simulink model "ControlePD_ind_pos"  (R2020a)
settings: Solver=FixedStepAuto  StartTime=0.0  StopTime=10  FixedStep=Ts
values from neighbouring files (symbols this model uses):
  Beff = 50    [controle.m]    (also in controle_FF.m; controle_PD.m)
  Jeff = 2.2    [controle.m]    (also in controle_FF.m = 0.5; controle_PD.m = 0.5)
  K = 17.7    [controle.m]    (also in controle_FF.m = 0.785398163397; controle_PD.m = 0.785398163397)
  Kd = (2*zeta*wn*Jeff - Beff)/K    (= -2.32768361582)    [controle.m]    (also in controle_FF.m = -44.5633840657; controle_PD.m = -44.5633840657)
  Kp = (wn^2*Jeff)/K    (= 0.497175141243)    [controle.m]    (also in controle_FF.m = 143.239448783; controle_PD.m = 143.239448783)
  N = 10    [controle.m]    (also in controle_FF.m = 3; controle_PD.m = 3)
  r = 1/100    (= 0.01)    [controle.m]    (also in controle_FF.m = 1./[231.22*4 139.138 139.138 231.22 231.22]; controle_PD.m = 1./[231.22*4 139.138 139.138 231.22 231.22])
  SP_theta = [0;0;0;0;0]    [controle.m]    (also in controle_FF.m = [0 0 0 0 0]; controle_PD.m)
settings Model: Creator=Karoline  LastModifiedBy=lunet
settings DataIOCC: ReturnWorkspaceOutputs=off
settings DebuggingCC: ArithmeticOperatorsInVariantConditions=warning
settings SFSimCC: SimUseLocalCustomCode=off  CustomCodeUndefinedFunction=UseInterfaceOnly
settings RTWCC: RTWUseLocalCustomCode=off
settings CodeAppCC: StateflowObjectComments=on

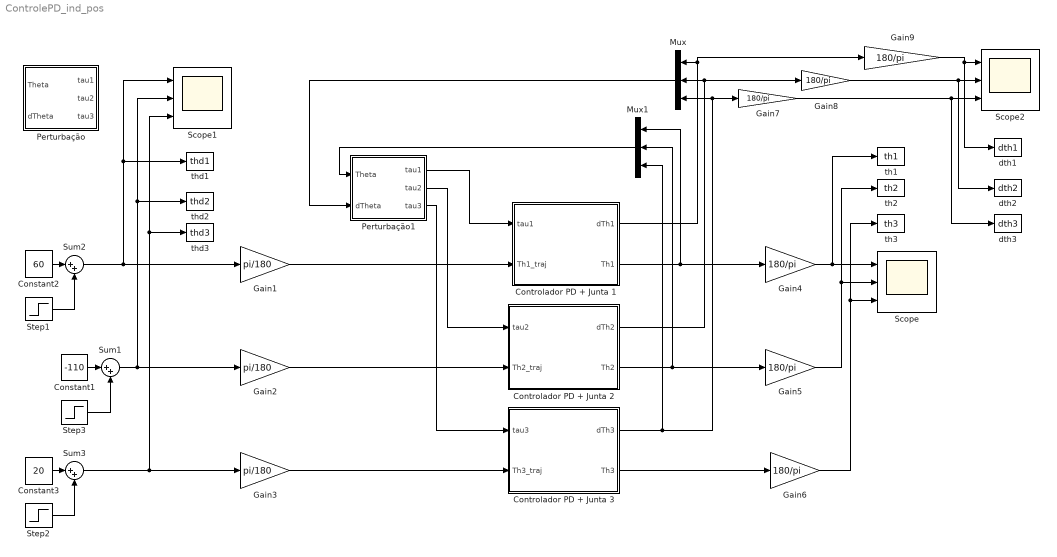
== system ControlePD_ind_pos ==
  Constant1 : Constant  Value=-110
  Constant2 : Constant  Value=60
  Constant3 : Constant  Value=20
  Controlador PD + Junta 1 : Subsystem
  Controlador PD + Junta 2 : Subsystem
  Controlador PD + Junta 3 : Subsystem
  Gain1 : Gain  Gain=pi/180
  Gain2 : Gain  Gain=pi/180
  Gain3 : Gain  Gain=pi/180
  Gain{4..9} (6 alike) : Gain  Gain=180/pi
  Mux : Mux  Inputs=3
  Mux1 : Mux  Inputs=3
  Perturbação : Subsystem
  Perturbação1 : Subsystem
  Scope : Scope  NumInputPorts=3
  Scope1 : Scope  NumInputPorts=3
  Scope2 : Scope  NumInputPorts=3
  Step1 : Step  Time=0  After=0  SampleTime=0
  Step2 : Step  Time=0  After=0  SampleTime=0
  Step3 : Step  Time=3  After=60  SampleTime=0
  Sum1 : Sum  Inputs=|++
  Sum2 : Sum  Inputs=|++
  Sum3 : Sum  Inputs=|++
  dth1 : ToWorkspace  VariableName=dth1  SampleTime=-1
  dth2 : ToWorkspace  VariableName=dth2  SampleTime=-1
  dth3 : ToWorkspace  VariableName=dth3  SampleTime=-1
  th1 : ToWorkspace  VariableName=th1  SampleTime=-1
  th2 : ToWorkspace  VariableName=th2  SampleTime=-1
  th3 : ToWorkspace  VariableName=th3  SampleTime=-1
  thd1 : ToWorkspace  VariableName=thd1  SampleTime=-1
  "thd2 " : ToWorkspace  VariableName=thd2  SampleTime=-1
  thd3 : ToWorkspace  VariableName=thd3  SampleTime=-1
  wires:
  Sum2/1 -> thd1/1, Scope1/1, Gain1/1
  Mux/1 -> Perturbação1/2(dTheta)
  Mux1/1 -> Perturbação1/1(Theta)
  Sum3/1 -> Scope1/3, thd3/1, Gain3/1
  Step3/1 -> Sum1/2
  Sum1/1 -> Scope1/2, "thd2 "/1, Gain2/1
  Constant1/1 -> Sum1/1
  Gain1/1 -> Controlador PD + Junta 1/2(Th1_traj)
  Gain2/1 -> Controlador PD + Junta 2/2(Th2_traj)
  Gain3/1 -> Controlador PD + Junta 3/2(Th3_traj)
  Gain4/1 -> th1/1, Scope/1
  Gain5/1 -> th2/1, Scope/2
  Gain6/1 -> th3/1, Scope/3
  Controlador PD + Junta 1/1("dTh1 ") -> Mux/1, Gain9/1
  Controlador PD + Junta 2/1("dTh2 ") -> Mux/2, Gain8/1
  Controlador PD + Junta 3/1("dTh3 ") -> Mux1/3, Mux/3, Gain7/1
  Controlador PD + Junta 1/2(Th1) -> Mux1/1, Gain4/1
  Controlador PD + Junta 2/2(Th2) -> Mux1/2, Gain5/1
  Controlador PD + Junta 3/2(Th3) -> Gain6/1
  Gain7/1 -> dth3/1, Scope2/3
  Gain8/1 -> dth2/1, Scope2/2
  Gain9/1 -> dth1/1, Scope2/1
  Step1/1 -> Sum2/2
  Constant2/1 -> Sum2/1
  Step2/1 -> Sum3/2
  Constant3/1 -> Sum3/1
  Perturbação1/1(tau1) -> Controlador PD + Junta 1/1(tau1)
  Perturbação1/2(tau2) -> Controlador PD + Junta 2/1(tau2)
  Perturbação1/3(tau3) -> Controlador PD + Junta 3/1(tau3)

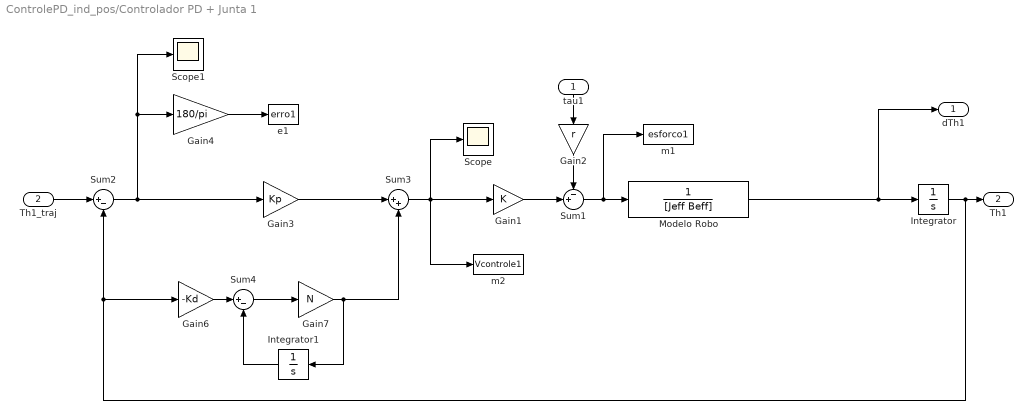
== system ControlePD_ind_pos/Controlador PD + Junta 1 ==
  tau1 : Inport
  Th1_traj : Inport  Port=2
  Gain1 : Gain  Gain=K
  Gain2 : Gain  Gain=r
  Gain3 : Gain  Gain=Kp
  Gain4 : Gain  Gain=180/pi
  Gain6 : Gain  Gain=-Kd
  Gain7 : Gain  Gain=N
  Integrator : Integrator  InitialCondition=SP_theta(1)*pi/180
  Integrator1 : Integrator
  Modelo Robo : TransferFcn  Denominator=[Jeff Beff]
  Scope : Scope
  Scope1 : Scope
  Sum1 : Sum  Inputs=-+|
  Sum2 : Sum  Inputs=|+-
  Sum3 : Sum  Inputs=|++
  Sum4 : Sum  Inputs=|+-
  e1 : ToWorkspace  VariableName=erro1  SampleTime=-1
  m1 : ToWorkspace  VariableName=esforco1  SampleTime=-1
  m2 : ToWorkspace  VariableName=Vcontrole1  SampleTime=-1
  "dTh1 " : Outport  VectorParamsAs1DForOutWhenUnconnected=off
  Th1 : Outport  Port=2  VectorParamsAs1DForOutWhenUnconnected=off
  wires:
  tau1/1 -> Gain2/1
  Gain1/1 -> Sum1/2
  Sum1/1 -> m1/1, Modelo Robo/1
  Integrator/1 -> Th1/1, Gain6/1, Sum2/2
  Th1_traj/1 -> Sum2/1
  Gain2/1 -> Sum1/1
  Gain4/1 -> e1/1
  Gain3/1 -> Sum3/1
  Sum3/1 -> m2/1, Scope/1, Gain1/1
  Modelo Robo/1 -> "dTh1 "/1, Integrator/1
  Gain7/1 -> Sum3/2, Integrator1/1
  Integrator1/1 -> Sum4/2
  Gain6/1 -> Sum4/1
  Sum4/1 -> Gain7/1
  Sum2/1 -> Gain3/1, Scope1/1, Gain4/1

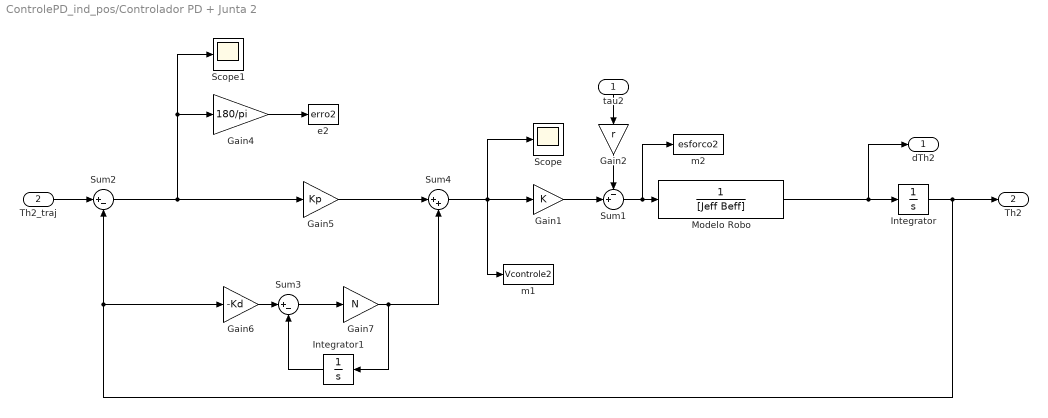
== system ControlePD_ind_pos/Controlador PD + Junta 2 ==
  tau2 : Inport
  Th2_traj : Inport  Port=2
  Gain1 : Gain  Gain=K
  Gain2 : Gain  Gain=r
  Gain4 : Gain  Gain=180/pi
  Gain5 : Gain  Gain=Kp
  Gain6 : Gain  Gain=-Kd
  Gain7 : Gain  Gain=N
  Integrator : Integrator  InitialCondition=SP_theta(2)*pi/180
  Integrator1 : Integrator
  "Modelo Robo " : TransferFcn  Denominator=[Jeff Beff]
  Scope : Scope
  Scope1 : Scope
  Sum1 : Sum  Inputs=-+|
  Sum2 : Sum  Inputs=|+-
  Sum3 : Sum  Inputs=|+-
  Sum4 : Sum  Inputs=|++
  e2 : ToWorkspace  VariableName=erro2  SampleTime=-1
  m1 : ToWorkspace  VariableName=Vcontrole2  SampleTime=-1
  m2 : ToWorkspace  VariableName=esforco2  SampleTime=-1
  "dTh2 " : Outport  VectorParamsAs1DForOutWhenUnconnected=off
  Th2 : Outport  Port=2  VectorParamsAs1DForOutWhenUnconnected=off
  wires:
  tau2/1 -> Gain2/1
  Gain1/1 -> Sum1/2
  Sum1/1 -> m2/1, "Modelo Robo "/1
  Th2_traj/1 -> Sum2/1
  Gain2/1 -> Sum1/1
  Gain4/1 -> e2/1
  Gain5/1 -> Sum4/1
  Sum4/1 -> m1/1, Scope/1, Gain1/1
  "Modelo Robo "/1 -> "dTh2 "/1, Integrator/1
  Sum2/1 -> Scope1/1, Gain4/1, Gain5/1
  Integrator1/1 -> Sum3/2
  Gain7/1 -> Sum4/2, Integrator1/1
  Integrator/1 -> Th2/1, Gain6/1, Sum2/2
  Sum3/1 -> Gain7/1
  Gain6/1 -> Sum3/1

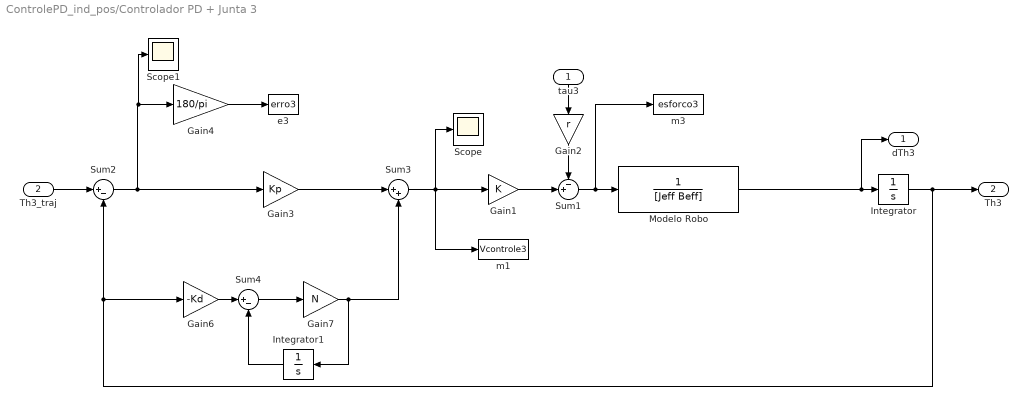
== system ControlePD_ind_pos/Controlador PD + Junta 3 ==
  tau3 : Inport
  Th3_traj : Inport  Port=2
  Gain1 : Gain  Gain=K
  Gain2 : Gain  Gain=r
  Gain3 : Gain  Gain=Kp
  Gain4 : Gain  Gain=180/pi
  Gain6 : Gain  Gain=-Kd
  Gain7 : Gain  Gain=N
  Integrator : Integrator  InitialCondition=SP_theta(3)*pi/180
  Integrator1 : Integrator
  Modelo Robo : TransferFcn  Denominator=[Jeff Beff]
  Scope : Scope
  Scope1 : Scope
  Sum1 : Sum  Inputs=-+|
  Sum2 : Sum  Inputs=|+-
  Sum3 : Sum  Inputs=|++
  Sum4 : Sum  Inputs=|+-
  e3 : ToWorkspace  VariableName=erro3  SampleTime=-1
  m1 : ToWorkspace  VariableName=Vcontrole3  SampleTime=-1
  m3 : ToWorkspace  VariableName=esforco3  SampleTime=-1
  "dTh3 " : Outport  VectorParamsAs1DForOutWhenUnconnected=off
  Th3 : Outport  Port=2  VectorParamsAs1DForOutWhenUnconnected=off
  wires:
  tau3/1 -> Gain2/1
  Gain1/1 -> Sum1/2
  Sum1/1 -> m3/1, Modelo Robo/1
  Th3_traj/1 -> Sum2/1
  Gain2/1 -> Sum1/1
  Gain4/1 -> e3/1
  Gain3/1 -> Sum3/1
  Sum3/1 -> m1/1, Scope/1, Gain1/1
  Modelo Robo/1 -> Integrator/1, "dTh3 "/1
  Sum2/1 -> Scope1/1, Gain4/1, Gain3/1
  Integrator1/1 -> Sum4/2
  Gain7/1 -> Sum3/2, Integrator1/1
  Integrator/1 -> Th3/1, Gain6/1, Sum2/2
  Sum4/1 -> Gain7/1
  Gain6/1 -> Sum4/1

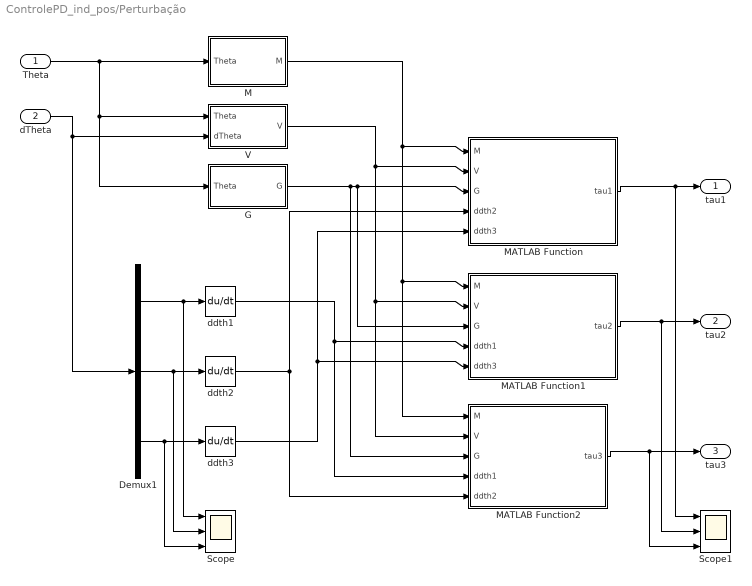
== system ControlePD_ind_pos/Perturbação ==
  Theta : Inport
  dTheta : Inport  Port=2
  Demux1 : Demux  Outputs=3
  G : Subsystem
  M : Subsystem
  MATLAB Function : MATLAB Function  TreatAsAtomicUnit=on
  MATLAB Function1 : MATLAB Function  TreatAsAtomicUnit=on
  MATLAB Function2 : MATLAB Function  TreatAsAtomicUnit=on
  Scope : Scope  NumInputPorts=3
  Scope1 : Scope  NumInputPorts=3
  V : Subsystem
  ddth1 : Derivative
  ddth2 : Derivative
  ddth3 : Derivative
  tau1 : Outport  VectorParamsAs1DForOutWhenUnconnected=off
  tau2 : Outport  Port=2  VectorParamsAs1DForOutWhenUnconnected=off
  tau3 : Outport  Port=3  VectorParamsAs1DForOutWhenUnconnected=off
  wires:
  dTheta/1 -> Demux1/1, V/2(dTheta)
  G/1(G) -> MATLAB Function2/3(G), MATLAB Function1/3(G), MATLAB Function/3(G)
  V/1(V) -> MATLAB Function/2(V), MATLAB Function1/2(V), MATLAB Function2/2(V)
  M/1(M) -> MATLAB Function2/1(M), MATLAB Function1/1(M), MATLAB Function/1(M)
  Theta/1 -> M/1(Theta), G/1(Theta), V/1(Theta)
  Demux1/1 -> Scope/1, ddth1/1
  Demux1/2 -> Scope/2, ddth2/1
  Demux1/3 -> Scope/3, ddth3/1
  ddth1/1 -> MATLAB Function2/4(ddth1), MATLAB Function1/4(ddth1)
  ddth3/1 -> MATLAB Function/5(ddth3), MATLAB Function1/5(ddth3)
  ddth2/1 -> MATLAB Function2/5(ddth2), MATLAB Function/4(ddth2)
  MATLAB Function/1(tau1) -> Scope1/1, tau1/1
  MATLAB Function1/1(tau2) -> Scope1/2, tau2/1
  MATLAB Function2/1(tau3) -> Scope1/3, tau3/1

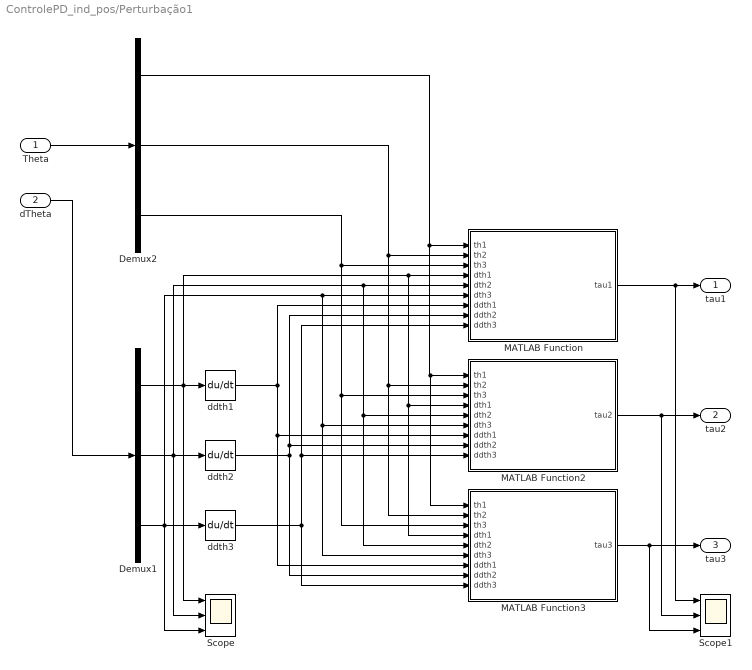
== system ControlePD_ind_pos/Perturbação1 ==
  Theta : Inport
  dTheta : Inport  Port=2
  Demux1 : Demux  Outputs=3
  Demux2 : Demux  Outputs=3
  MATLAB Function : MATLAB Function  TreatAsAtomicUnit=on
  MATLAB Function2 : MATLAB Function  TreatAsAtomicUnit=on
  MATLAB Function3 : MATLAB Function  TreatAsAtomicUnit=on
  Scope : Scope  NumInputPorts=3
  Scope1 : Scope  NumInputPorts=3
  ddth1 : Derivative
  ddth2 : Derivative
  ddth3 : Derivative
  tau1 : Outport  VectorParamsAs1DForOutWhenUnconnected=off
  tau2 : Outport  Port=2  VectorParamsAs1DForOutWhenUnconnected=off
  tau3 : Outport  Port=3  VectorParamsAs1DForOutWhenUnconnected=off
  wires:
  dTheta/1 -> Demux1/1
  Demux1/1 -> MATLAB Function3/4(dth1), MATLAB Function2/4(dth1), MATLAB Function/4(dth1), Scope/1, ddth1/1
  Demux1/2 -> MATLAB Function3/5(dth2), MATLAB Function2/5(dth2), MATLAB Function/5(dth2), Scope/2, ddth2/1
  Demux1/3 -> MATLAB Function3/6(dth3), MATLAB Function2/6(dth3), MATLAB Function/6(dth3), Scope/3, ddth3/1
  ddth1/1 -> MATLAB Function3/7(ddth1), MATLAB Function2/7(ddth1), MATLAB Function/7(ddth1)
  ddth3/1 -> MATLAB Function3/9(ddth3), MATLAB Function2/9(ddth3), MATLAB Function/9(ddth3)
  ddth2/1 -> MATLAB Function3/8(ddth2), MATLAB Function2/8(ddth2), MATLAB Function/8(ddth2)
  MATLAB Function/1(tau1) -> tau1/1, Scope1/1
  MATLAB Function2/1(tau2) -> tau2/1, Scope1/2
  MATLAB Function3/1(tau3) -> tau3/1, Scope1/3
  Theta/1 -> Demux2/1
  Demux2/3 -> MATLAB Function3/3(th3), MATLAB Function2/3(th3), MATLAB Function/3(th3)
  Demux2/2 -> MATLAB Function3/2(th2), MATLAB Function2/2(th2), MATLAB Function/2(th2)
  Demux2/1 -> MATLAB Function3/1(th1), MATLAB Function2/1(th1), MATLAB Function/1(th1)

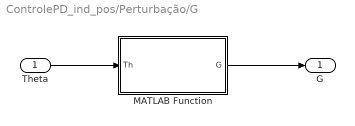
== system ControlePD_ind_pos/Perturbação/G ==
  Theta : Inport
  MATLAB Function : MATLAB Function  TreatAsAtomicUnit=on
  G : Outport  VectorParamsAs1DForOutWhenUnconnected=off
  wires:
  Theta/1 -> MATLAB Function/1(Th)
  MATLAB Function/1(G) -> G/1

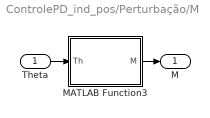
== system ControlePD_ind_pos/Perturbação/M ==
  Theta : Inport
  MATLAB Function3 : MATLAB Function  TreatAsAtomicUnit=on
  M : Outport  VectorParamsAs1DForOutWhenUnconnected=off
  wires:
  Theta/1 -> MATLAB Function3/1(Th)
  MATLAB Function3/1(M) -> M/1

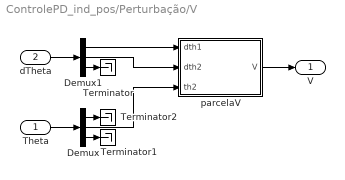
== system ControlePD_ind_pos/Perturbação/V ==
  Theta : Inport
  dTheta : Inport  Port=2
  Demux : Demux  Outputs=3
  Demux1 : Demux  Outputs=3
  Terminator : Terminator
  Terminator1 : Terminator
  Terminator2 : Terminator
  parcelaV : MATLAB Function  TreatAsAtomicUnit=on
  V : Outport  VectorParamsAs1DForOutWhenUnconnected=off
  wires:
  Theta/1 -> Demux/1
  dTheta/1 -> Demux1/1
  Demux1/1 -> parcelaV/1(dth1)
  Demux1/2 -> parcelaV/2(dth2)
  Demux/2 -> parcelaV/3(th2)
  parcelaV/1(V) -> V/1
  Demux1/3 -> Terminator/1
  Demux/1 -> Terminator2/1
  Demux/3 -> Terminator1/1

== matlab function ControlePD_ind_pos/Perturbação1/MATLAB Function ==
  data: th1 input; th2 input; tau1 output; th3 input; dth1 input; dth2 input; dth3 input; ddth1 input; ddth2 input; ddth3 input
function tau1  = calcul_dk1(th1,th2,th3,dth1,dth2,dth3,ddth1,ddth2,ddth3)

I1 = 1;
I2 = 1;
I3 = 1;
m1 = 1;
m2 = 1;
m3 = 1;
Lc1 = 0.05;
Lc2 = 0.05;
Lc3 = 0.05;
g = 9.81;

tau1 = I1*ddth1 + I2*ddth1*cos(th2)^2 + I2*ddth1*sin(th2)^2 + I3*ddth1*cos(th2)^2*cos(th3)^2 + I3*ddth1*cos(th2)^2*sin(th3)^2 + I3*ddth1*cos(th3)^2*sin(th2)^2 + I3*ddth1*sin(th2)^2*sin(th3)^2 + (ddth1*m3*cos(th1)^2*cos(th2)^2)/25 + (ddth1*m3*cos(th2)^2*sin(th1)^2)/25 + Lc2^2*ddth1*m2*cos(th1)^2*cos(th2)^2 + Lc2^2*ddth1*m2*cos(th2)^2*sin(th1)^2 - (2*dth1*dth2*m3*cos(th1)^2*cos(th2)*sin(th2))/25 + Lc3^2*ddth1*m3*cos(th1)^2*cos(th2)^2*sin(th3)^2 + Lc3^2*ddth1*m3*cos(th1)^2*cos(th3)^2*sin(th2)^2 - (2*dth1*dth2*m3*cos(th2)*sin(th1)^2*sin(th2))/25 + Lc3^2*ddth1*m3*cos(th2)^2*sin(th1)^2*sin(th3)^2 + Lc3^2*ddth1*m3*cos(th3)^2*sin(th1)^2*sin(th2)^2 - (2*Lc3*ddth1*m3*cos(th1)^2*cos(th2)^2*sin(th3))/5 - (2*Lc3*ddth1*m3*cos(th2)^2*sin(th1)^2*sin(th3))/5 - (2*Lc3*dth1*dth2*m3*cos(th1)^2*cos(th2)^2*cos(th3))/5 - (2*Lc3*dth1*dth3*m3*cos(th1)^2*cos(th2)^2*cos(th3))/5 - 2*Lc2^2*dth1*dth2*m2*cos(th1)^2*cos(th2)*sin(th2) + (2*Lc3*dth1*dth2*m3*cos(th1)^2*cos(th3)*sin(th2)^2)/5 - (2*Lc3*dth1*dth2*m3*cos(th2)^2*cos(th3)*sin(th1)^2)/5 - (2*Lc3*dth1*dth3*m3*cos(th2)^2*cos(th3)*sin(th1)^2)/5 - 2*Lc2^2*dth1*dth2*m2*cos(th2)*sin(th1)^2*sin(th2) + (2*Lc3*dth1*dth2*m3*cos(th3)*sin(th1)^2*sin(th2)^2)/5 - (2*Lc3*ddth1*m3*cos(th1)^2*cos(th2)*cos(th3)*sin(th2))/5 - (2*Lc3*ddth1*m3*cos(th2)*cos(th3)*sin(th1)^2*sin(th2))/5 + 2*Lc3^2*dth1*dth2*m3*cos(th1)^2*cos(th2)*cos(th3)^2*sin(th2) + 2*Lc3^2*dth1*dth2*m3*cos(th1)^2*cos(th2)^2*cos(th3)*sin(th3) + 2*Lc3^2*dth1*dth3*m3*cos(th1)^2*cos(th2)*cos(th3)^2*sin(th2) + 2*Lc3^2*dth1*dth3*m3*cos(th1)^2*cos(th2)^2*cos(th3)*sin(th3) + 2*Lc3^2*dth1*dth2*m3*cos(th2)*cos(th3)^2*sin(th1)^2*sin(th2) - 2*Lc3^2*dth1*dth2*m3*cos(th1)^2*cos(th2)*sin(th2)*sin(th3)^2 - 2*Lc3^2*dth1*dth2*m3*cos(th1)^2*cos(th3)*sin(th2)^2*sin(th3) + 2*Lc3^2*dth1*dth2*m3*cos(th2)^2*cos(th3)*sin(th1)^2*sin(th3) + 2*Lc3^2*dth1*dth3*m3*cos(th2)*cos(th3)^2*sin(th1)^2*sin(th2) - 2*Lc3^2*dth1*dth3*m3*cos(th1)^2*cos(th2)*sin(th2)*sin(th3)^2 - 2*Lc3^2*dth1*dth3*m3*cos(th1)^2*cos(th3)*sin(th2)^2*sin(th3) + 2*Lc3^2*dth1*dth3*m3*cos(th2)^2*cos(th3)*sin(th1)^2*sin(th3) - 2*Lc3^2*dth1*dth2*m3*cos(th2)*sin(th1)^2*sin(th2)*sin(th3)^2 - 2*Lc3^2*dth1*dth2*m3*cos(th3)*sin(th1)^2*sin(th2)^2*sin(th3) - 2*Lc3^2*dth1*dth3*m3*cos(th2)*sin(th1)^2*sin(th2)*sin(th3)^2 - 2*Lc3^2*dth1*dth3*m3*cos(th3)*sin(th1)^2*sin(th2)^2*sin(th3) + 2*Lc3^2*ddth1*m3*cos(th1)^2*cos(th2)*cos(th3)*sin(th2)*sin(th3) + 2*Lc3^2*ddth1*m3*cos(th2)*cos(th3)*sin(th1)^2*sin(th2)*sin(th3) + (4*Lc3*dth1*dth2*m3*cos(th1)^2*cos(th2)*sin(th2)*sin(th3))/5 + (2*Lc3*dth1*dth3*m3*cos(th1)^2*cos(th2)*sin(th2)*sin(th3))/5 + (4*Lc3*dth1*dth2*m3*cos(th2)*sin(th1)^2*sin(th2)*sin(th3))/5 + (2*Lc3*dth1*dth3*m3*cos(th2)*sin(th1)^2*sin(th2)*sin(th3))/5;

== matlab function ControlePD_ind_pos/Perturbação1/MATLAB Function2 ==
  data: th1 input; th2 input; tau2 output; th3 input; dth1 input; dth2 input; dth3 input; ddth1 input; ddth2 input; ddth3 input
function tau2  = calcul_dk2(th1,th2,th3,dth1,dth2,dth3,ddth1,ddth2,ddth3)

I1 = 1;
I2 = 1;
I3 = 1;
m1 = 1;
m2 = 1;
m3 = 1;
Lc1 = 0.05;
Lc2 = 0.05;
Lc3 = 0.05;
g = 9.81;

tau2 =   I2*ddth2 + I3*ddth2 + I3*ddth3 + Lc2^2*ddth2*m2*cos(th2)^2 - Lc3*g*m3*sin(th2 + th3) + Lc2*g*m2*cos(th2) + (ddth2*m3*cos(th2 + th3)^2*cos(th3)^2)/25 + (ddth2*m3*sin(th2 + th3)^2*sin(th3)^2)/25 + Lc3^2*ddth2*m3*sin(th2 + th3)^2 + Lc3^2*ddth3*m3*sin(th2 + th3)^2 + Lc3^2*ddth2*m3*cos(th2 + th3)^2*cos(th1)^2 + Lc3^2*ddth3*m3*cos(th2 + th3)^2*cos(th1)^2 - (dth2^2*m3*cos(th2 + th3)*sin(th2 + th3)*cos(th3)^2)/25 + Lc3^2*ddth2*m3*cos(th2 + th3)^2*sin(th1)^2 + Lc3^2*ddth3*m3*cos(th2 + th3)^2*sin(th1)^2 + (dth2^2*m3*cos(th2 + th3)*sin(th2 + th3)*sin(th3)^2)/25 + (dth2^2*m3*cos(th2 + th3)^2*cos(th3)*sin(th3))/25 + Lc2^2*ddth2*m2*cos(th1)^2*sin(th2)^2 - (dth2^2*m3*sin(th2 + th3)^2*cos(th3)*sin(th3))/25 + Lc2^2*ddth2*m2*sin(th1)^2*sin(th2)^2 - (2*Lc3*ddth2*m3*sin(th2 + th3)^2*sin(th3))/5 - (Lc3*ddth3*m3*sin(th2 + th3)^2*sin(th3))/5 - (dth1^2*m3*cos(th1)^2*cos(th2)*sin(th2))/25 - (dth1^2*m3*cos(th2)*sin(th1)^2*sin(th2))/25 + Lc3^2*dth2^2*m3*cos(th2 + th3)*sin(th2 + th3) + Lc3^2*dth3^2*m3*cos(th2 + th3)*sin(th2 + th3) + (ddth2*m3*cos(th2 + th3)^2*cos(th1)^2*sin(th3)^2)/25 + (ddth2*m3*sin(th2 + th3)^2*cos(th1)^2*cos(th3)^2)/25 - (Lc3*dth2^2*m3*cos(th2 + th3)^2*cos(th3))/5 + (ddth2*m3*cos(th2 + th3)^2*sin(th1)^2*sin(th3)^2)/25 + (ddth2*m3*sin(th2 + th3)^2*cos(th3)^2*sin(th1)^2)/25 + (Lc3*dth2^2*m3*sin(th2 + th3)^2*cos(th3))/5 - (Lc3*dth3^2*m3*sin(th2 + th3)^2*cos(th3))/5 - 3*Lc2^2*dth2^2*m2*cos(th2)*sin(th2) + (Lc3*dth2^2*m3*cos(th2 + th3)^2*cos(th3)*sin(th1)^2)/5 - (Lc3*dth2^2*m3*sin(th2 + th3)^2*cos(th1)^2*cos(th3))/5 - (Lc3*dth3^2*m3*cos(th2 + th3)^2*cos(th3)*sin(th1)^2)/5 + (2*dth2*m3*cos(th2 + th3)*sin(th2 + th3)*sin(th3)^2*(dth2 + dth3))/25 - (Lc3*dth2^2*m3*sin(th2 + th3)^2*cos(th3)*sin(th1)^2)/5 - (Lc3*dth1^2*m3*cos(th1)^2*cos(th2)^2*cos(th3))/5 + (2*dth2*m3*cos(th2 + th3)^2*cos(th3)*sin(th3)*(dth2 + dth3))/25 - (2*Lc3*dth2^2*m3*cos(th2 + th3)*sin(th2 + th3)*sin(th3))/5 + (Lc3*dth3^2*m3*cos(th2 + th3)*sin(th2 + th3)*sin(th3))/5 - Lc2^2*dth1^2*m2*cos(th1)^2*cos(th2)*sin(th2) + 3*Lc2^2*dth2^2*m2*cos(th1)^2*cos(th2)*sin(th2) + (Lc3*dth1^2*m3*cos(th1)^2*cos(th3)*sin(th2)^2)/5 - (Lc3*dth1^2*m3*cos(th2)^2*cos(th3)*sin(th1)^2)/5 + (2*dth2*dth3*m3*cos(th2 + th3)*sin(th2 + th3)*cos(th3)^2)/25 - (2*dth2*m3*sin(th2 + th3)^2*cos(th3)*sin(th3)*(dth2 + dth3))/25 - Lc2^2*dth1^2*m2*cos(th2)*sin(th1)^2*sin(th2) + 3*Lc2^2*dth2^2*m2*cos(th2)*sin(th1)^2*sin(th2) + (Lc3*dth1^2*m3*cos(th3)*sin(th1)^2*sin(th2)^2)/5 - (2*dth2*dth3*m3*cos(th2 + th3)*sin(th2 + th3)*sin(th3)^2)/25 + (2*ddth2*m3*cos(th2 + th3)*sin(th2 + th3)*cos(th3)*sin(th3))/25 - (2*dth2*dth3*m3*cos(th2 + th3)^2*cos(th3)*sin(th3))/25 + (dth2^2*m3*cos(th2 + th3)*sin(th2 + th3)*cos(th1)^2*cos(th3)^2)/25 + 2*Lc3^2*dth2*m3*cos(th2 + th3)*sin(th2 + th3)*(dth2 + dth3) + 2*Lc3^2*dth3*m3*cos(th2 + th3)*sin(th2 + th3)*(dth2 + dth3) + (2*dth2*dth3*m3*sin(th2 + th3)^2*cos(th3)*sin(th3))/25 - (dth2^2*m3*cos(th2 + th3)*sin(th2 + th3)*cos(th1)^2*sin(th3)^2)/25 + (dth2^2*m3*cos(th2 + th3)*sin(th2 + th3)*cos(th3)^2*sin(th1)^2)/25 - (dth2^2*m3*cos(th2 + th3)*sin(th2 + th3)*sin(th1)^2*sin(th3)^2)/25 - (2*Lc3*dth2*m3*cos(th2 + th3)^2*cos(th3)*(dth2 + dth3))/5 - (Lc3*dth3*m3*cos(th2 + th3)^2*cos(th3)*(dth2 + dth3))/5 - (dth2^2*m3*cos(th2 + th3)^2*cos(th1)^2*cos(th3)*sin(th3))/25 + (2*Lc3*dth2*m3*sin(th2 + th3)^2*cos(th3)*(dth2 + dth3))/5 + (Lc3*dth3*m3*sin(th2 + th3)^2*cos(th3)*(dth2 + dth3))/5 - (dth2^2*m3*cos(th2 + th3)^2*cos(th3)*sin(th1)^2*sin(th3))/25 + (dth2^2*m3*sin(th2 + th3)^2*cos(th1)^2*cos(th3)*sin(th3))/25 - (2*Lc3*ddth2*m3*cos(th2 + th3)^2*cos(th1)^2*sin(th3))/5 - (Lc3*ddth3*m3*cos(th2 + th3)^2*cos(th1)^2*sin(th3))/5 + 2*Lc3^2*dth2*dth3*m3*cos(th2 + th3)*sin(th2 + th3) + (dth2^2*m3*sin(th2 + th3)^2*cos(th3)*sin(th1)^2*sin(th3))/25 - (2*Lc3*ddth2*m3*cos(th2 + th3)^2*sin(th1)^2*sin(th3))/5 - (Lc3*ddth3*m3*cos(th2 + th3)^2*sin(th1)^2*sin(th3))/5 - (2*Lc3*ddth2*m3*cos(th2 + th3)*sin(th2 + th3)*cos(th3))/5 - (Lc3*ddth3*m3*cos(th2 + th3)*sin(th2 + th3)*cos(th3))/5 - (Lc3*dth2*dth3*m3*cos(th2 + th3)^2*cos(th3))/5 - (Lc3*dth2*dth3*m3*sin(th2 + th3)^2*cos(th3))/5 - Lc3^2*dth2^2*m3*cos(th2 + th3)*sin(th2 + th3)*cos(th1)^2 - Lc3^2*dth3^2*m3*cos(th2 + th3)*sin(th2 + th3)*cos(th1)^2 - Lc3^2*dth2^2*m3*cos(th2 + th3)*sin(th2 + th3)*sin(th1)^2 - Lc3^2*dth3^2*m3*cos(th2 + th3)*sin(th2 + th3)*sin(th1)^2 + (Lc3*dth2^2*m3*cos(th2 + th3)^2*cos(th1)^2*cos(th3))/5 - (Lc3*dth3^2*m3*cos(th2 + th3)^2*cos(th1)^2*cos(th3))/5 - (2*dth2*m3*cos(th2 + th3)*sin(th2 + th3)*cos(th3)^2*(dth2 + dth3))/25 + (2*Lc3*ddth2*m3*cos(th2 + th3)*sin(th2 + th3)*cos(th3)*sin(th1)^2)/5 + (Lc3*ddth3*m3*cos(th2 + th3)*sin(th2 + th3)*cos(th3)*sin(th1)^2)/5 - (Lc3*dth2*dth3*m3*cos(th2 + th3)^2*cos(th3)*sin(th1)^2)/5 - (Lc3*dth2*dth3*m3*sin(th2 + th3)^2*cos(th1)^2*cos(th3))/5 - (Lc3*dth2*dth3*m3*sin(th2 + th3)^2*cos(th3)*sin(th1)^2)/5 + (2*dth2*m3*cos(th2 + th3)*sin(th2 + th3)*cos(th1)^2*cos(th3)^2*(dth2 + dth3))/25 - (2*dth2*m3*cos(th2 + th3)*sin(th2 + th3)*cos(th1)^2*sin(th3)^2*(dth2 + dth3))/25 + (2*dth2*m3*cos(th2 + th3)*sin(th2 + th3)*cos(th3)^2*sin(th1)^2*(dth2 + dth3))/25 - (2*dth2*m3*cos(th2 + th3)*sin(th2 + th3)*sin(th1)^2*sin(th3)^2*(dth2 + dth3))/25 - (2*dth2*m3*cos(th2 + th3)^2*cos(th1)^2*cos(th3)*sin(th3)*(dth2 + dth3))/25 + (2*Lc3*dth2^2*m3*cos(th2 + th3)*sin(th2 + th3)*cos(th1)^2*sin(th3))/5 - (Lc3*dth3^2*m3*cos(th2 + th3)*sin(th2 + th3)*cos(th1)^2*sin(th3))/5 + Lc3^2*dth1^2*m3*cos(th1)^2*cos(th2)*cos(th3)^2*sin(th2) + Lc3^2*dth1^2*m3*cos(th1)^2*cos(th2)^2*cos(th3)*sin(th3) - (2*dth2*dth3*m3*cos(th2 + th3)*sin(th2 + th3)*cos(th1)^2*cos(th3)^2)/25 - (2*dth2*m3*cos(th2 + th3)^2*cos(th3)*sin(th1)^2*sin(th3)*(dth2 + dth3))/25 + (2*dth2*m3*sin(th2 + th3)^2*cos(th1)^2*cos(th3)*sin(th3)*(dth2 + dth3))/25 + (2*Lc3*dth2^2*m3*cos(th2 + th3)*sin(th2 + th3)*sin(th1)^2*sin(th3))/5 - (Lc3*dth3^2*m3*cos(th2 + th3)*sin(th2 + th3)*sin(th1)^2*sin(th3))/5 + Lc3^2*dth1^2*m3*cos(th2)*cos(th3)^2*sin(th1)^2*sin(th2) - Lc3^2*dth1^2*m3*cos(th1)^2*cos(th2)*sin(th2)*sin(th3)^2 - Lc3^2*dth1^2*m3*cos(th1)^2*cos(th3)*sin(th2)^2*sin(th3) + Lc3^2*dth1^2*m3*cos(th2)^2*cos(th3)*sin(th1)^2*sin(th3) + (2*dth2*dth3*m3*cos(th2 + th3)*sin(th2 + th3)*cos(th1)^2*sin(th3)^2)/25 - (2*dth2*dth3*m3*cos(th2 + th3)*sin(th2 + th3)*cos(th3)^2*sin(th1)^2)/25 + (2*dth2*m3*sin(th2 + th3)^2*cos(th3)*sin(th1)^2*sin(th3)*(dth2 + dth3))/25 - Lc3^2*dth1^2*m3*cos(th2)*sin(th1)^2*sin(th2)*sin(th3)^2 - Lc3^2*dth1^2*m3*cos(th3)*sin(th1)^2*sin(th2)^2*sin(th3) + (2*dth2*dth3*m3*cos(th2 + th3)*sin(th2 + th3)*sin(th1)^2*sin(th3)^2)/25 - (2*ddth2*m3*cos(th2 + th3)*sin(th2 + th3)*cos(th1)^2*cos(th3)*sin(th3))/25 + (2*dth2*dth3*m3*cos(th2 + th3)^2*cos(th1)^2*cos(th3)*sin(th3))/25 - (2*ddth2*m3*cos(th2 + th3)*sin(th2 + th3)*cos(th3)*sin(th1)^2*sin(th3))/25 - 2*Lc3^2*dth2*m3*cos(th2 + th3)*sin(th2 + th3)*cos(th1)^2*(dth2 + dth3) - 2*Lc3^2*dth3*m3*cos(th2 + th3)*sin(th2 + th3)*cos(th1)^2*(dth2 + dth3) + (2*dth2*dth3*m3*cos(th2 + th3)^2*cos(th3)*sin(th1)^2*sin(th3))/25 - (2*dth2*dth3*m3*sin(th2 + th3)^2*cos(th1)^2*cos(th3)*sin(th3))/25 - 2*Lc3^2*dth2*m3*cos(th2 + th3)*sin(th2 + th3)*sin(th1)^2*(dth2 + dth3) - 2*Lc3^2*dth3*m3*cos(th2 + th3)*sin(th2 + th3)*sin(th1)^2*(dth2 + dth3) - (2*dth2*dth3*m3*sin(th2 + th3)^2*cos(th3)*sin(th1)^2*sin(th3))/25 + (2*Lc3*dth1^2*m3*cos(th1)^2*cos(th2)*sin(th2)*sin(th3))/5 + (2*Lc3*dth2*m3*cos(th2 + th3)^2*cos(th1)^2*cos(th3)*(dth2 + dth3))/5 + (Lc3*dth3*m3*cos(th2 + th3)^2*cos(th1)^2*cos(th3)*(dth2 + dth3))/5 + (2*Lc3*dth1^2*m3*cos(th2)*sin(th1)^2*sin(th2)*sin(th3))/5 + (2*Lc3*dth2*m3*cos(th2 + th3)^2*cos(th3)*sin(th1)^2*(dth2 + dth3))/5 - (2*Lc3*dth2*m3*sin(th2 + th3)^2*cos(th1)^2*cos(th3)*(dth2 + dth3))/5 + (Lc3*dth3*m3*cos(th2 + th3)^2*cos(th3)*sin(th1)^2*(dth2 + dth3))/5 - (Lc3*dth3*m3*sin(th2 + th3)^2*cos(th1)^2*cos(th3)*(dth2 + dth3))/5 - 2*Lc3^2*dth2*dth3*m3*cos(th2 + th3)*sin(th2 + th3)*cos(th1)^2 - (2*Lc3*dth2*m3*sin(th2 + th3)^2*cos(th3)*sin(th1)^2*(dth2 + dth3))/5 - (Lc3*dth3*m3*sin(th2 + th3)^2*cos(th3)*sin(th1)^2*(dth2 + dth3))/5 - 2*Lc3^2*dth2*dth3*m3*cos(th2 + th3)*sin(th2 + th3)*sin(th1)^2 + (2*Lc3*ddth2*m3*cos(th2 + th3)*sin(th2 + th3)*cos(th1)^2*cos(th3))/5 + (Lc3*ddth3*m3*cos(th2 + th3)*sin(th2 + th3)*cos(th1)^2*cos(th3))/5 - (4*Lc3*dth2*m3*cos(th2 + th3)*sin(th2 + th3)*sin(th3)*(dth2 + dth3))/5 - (2*Lc3*dth3*m3*cos(th2 + th3)*sin(th2 + th3)*sin(th3)*(dth2 + dth3))/5 - (Lc3*dth2*dth3*m3*cos(th2 + th3)^2*cos(th1)^2*cos(th3))/5 + (4*Lc3*dth2*m3*cos(th2 + th3)*sin(th2 + th3)*cos(th1)^2*sin(th3)*(dth2 + dth3))/5 + (2*Lc3*dth3*m3*cos(th2 + th3)*sin(th2 + th3)*cos(th1)^2*sin(th3)*(dth2 + dth3))/5 + (4*Lc3*dth2*m3*cos(th2 + th3)*sin(th2 + th3)*sin(th1)^2*sin(th3)*(dth2 + dth3))/5 + (2*Lc3*dth3*m3*cos(th2 + th3)*sin(th2 + th3)*sin(th1)^2*sin(th3)*(dth2 + dth3))/5;

== matlab function ControlePD_ind_pos/Perturbação/G/MATLAB Function ==
  data: Th input; G output
function G = calcul_G(Th)

th1 = Th(1);
th2 = Th(2);
th3 = Th(3);

G = [(1617*cos(th1 + th2))/100 + (3871*cos(th1))/100;...
    (1617*cos(th1 + th2))/100;...
    0];

== matlab function ControlePD_ind_pos/Perturbação/MATLAB Function1 ==
  data: M input; V input; tau2 output; G input; ddth1 input; ddth3 input
function tau2  = calcul_dk2(M,V,G,ddth1, ddth3)


% tau2 = m21*ddth1 + m23*ddth3 + v2 + g2;
tau2 = M(2,1)*ddth1 + M(2,3)*ddth3 + V(2,1) + G(2);

== matlab function ControlePD_ind_pos/Perturbação/MATLAB Function ==
  data: M input; V input; tau1 output; G input; ddth2 input; ddth3 input
function tau1  = calcul_dk1(M,V,G,ddth2,ddth3)


% tau1 = m12*ddth2 + m13*ddth3 + v1 + g1;
tau1 = M(1,2)*ddth2 + M(1,3)*ddth3 + V(1,1) + G(1);

== matlab function ControlePD_ind_pos/Perturbação/MATLAB Function2 ==
  data: M input; V input; tau3 output; G input; ddth1 input; ddth2 input
function tau3  = calcul_dk3(M, V, G, ddth1, ddth2)



% tau3 = m31*ddth1 + m32*ddth2 + v3 + g3;
tau3 = M(3,1)*ddth1 + M(3,2)*ddth2 + V(3,1) + G(3);

== matlab function ControlePD_ind_pos/Perturbação/M/MATLAB Function3 ==
  data: Th input; M output
function M = calcul_M(Th)

th1 = Th(1);
th2 = Th(2);
th3 = Th(3);

M = [(33*cos(th2))/20 + 29/10, (33*cos(th2))/40 + 37/40, 1/10;...
     (33*cos(th2))/40 + 37/40,                    37/40, 1/10;...
                         1/10,                     1/10, 1/10];

== matlab function ControlePD_ind_pos/Perturbação/V/parcelaV ==
  data: dth1 input; V output; dth2 input; th2 input
function V = parcelaV(dth1,dth2,th2)
%#codegen

%    This function was generated by the Symbolic Math Toolbox version 8.2.
%    18-Oct-2019 15:37:48

t2 = sin(th2);
V = [dth2.^2.*t2.*(-3.3e1./4.0e1)-dth1.*dth2.*t2.*(3.3e1./2.0e1);dth1.^2.*t2.*(3.3e1./4.0e1);0.0];

== matlab function ControlePD_ind_pos/Perturbação1/MATLAB Function3 ==
  data: th1 input; th2 input; tau3 output; th3 input; dth1 input; dth2 input; dth3 input; ddth1 input; ddth2 input; ddth3 input
function tau3  = calcul_dk3(th1,th2,th3,dth1,dth2,dth3,ddth1,ddth2,ddth3)

I1 = 1;
I2 = 1;
I3 = 1;
m1 = 1;
m2 = 1;
m3 = 1;
Lc1 = 0.05;
Lc2 = 0.05;
Lc3 = 0.05;
g = 9.81;

tau3 = I3*ddth2 + I3*ddth3 - Lc3*g*m3*sin(th2 + th3) + Lc3^2*ddth2*m3*sin(th2 + th3)^2 + Lc3^2*ddth3*m3*sin(th2 + th3)^2 + Lc3^2*ddth2*m3*cos(th2 + th3)^2*cos(th1)^2 + Lc3^2*ddth3*m3*cos(th2 + th3)^2*cos(th1)^2 + Lc3^2*ddth2*m3*cos(th2 + th3)^2*sin(th1)^2 + Lc3^2*ddth3*m3*cos(th2 + th3)^2*sin(th1)^2 - (Lc3*ddth2*m3*sin(th2 + th3)^2*sin(th3))/5 + Lc3^2*dth2^2*m3*cos(th2 + th3)*sin(th2 + th3) + Lc3^2*dth3^2*m3*cos(th2 + th3)*sin(th2 + th3) - (Lc3*dth2^2*m3*cos(th2 + th3)^2*cos(th3))/5 - (Lc3*dth2^2*m3*sin(th2 + th3)^2*cos(th1)^2*cos(th3))/5 - (Lc3*dth2^2*m3*sin(th2 + th3)^2*cos(th3)*sin(th1)^2)/5 - (Lc3*dth1^2*m3*cos(th1)^2*cos(th2)^2*cos(th3))/5 - (Lc3*dth2^2*m3*cos(th2 + th3)*sin(th2 + th3)*sin(th3))/5 - (Lc3*dth1^2*m3*cos(th2)^2*cos(th3)*sin(th1)^2)/5 + 2*Lc3^2*dth2*m3*cos(th2 + th3)*sin(th2 + th3)*(dth2 + dth3) + 2*Lc3^2*dth3*m3*cos(th2 + th3)*sin(th2 + th3)*(dth2 + dth3) - (Lc3*dth2*m3*cos(th2 + th3)^2*cos(th3)*(dth2 + dth3))/5 + (Lc3*dth2*m3*sin(th2 + th3)^2*cos(th3)*(dth2 + dth3))/5 - (Lc3*ddth2*m3*cos(th2 + th3)^2*cos(th1)^2*sin(th3))/5 + 2*Lc3^2*dth2*dth3*m3*cos(th2 + th3)*sin(th2 + th3) - (Lc3*ddth2*m3*cos(th2 + th3)^2*sin(th1)^2*sin(th3))/5 - (Lc3*ddth2*m3*cos(th2 + th3)*sin(th2 + th3)*cos(th3))/5 - (Lc3*dth2*dth3*m3*cos(th2 + th3)^2*cos(th3))/5 - (Lc3*dth2*dth3*m3*sin(th2 + th3)^2*cos(th3))/5 - Lc3^2*dth2^2*m3*cos(th2 + th3)*sin(th2 + th3)*cos(th1)^2 - Lc3^2*dth3^2*m3*cos(th2 + th3)*sin(th2 + th3)*cos(th1)^2 - Lc3^2*dth2^2*m3*cos(th2 + th3)*sin(th2 + th3)*sin(th1)^2 - Lc3^2*dth3^2*m3*cos(th2 + th3)*sin(th2 + th3)*sin(th1)^2 + (Lc3*ddth2*m3*cos(th2 + th3)*sin(th2 + th3)*cos(th3)*sin(th1)^2)/5 - (Lc3*dth2*dth3*m3*cos(th2 + th3)^2*cos(th3)*sin(th1)^2)/5 - (Lc3*dth2*dth3*m3*sin(th2 + th3)^2*cos(th1)^2*cos(th3))/5 - (Lc3*dth2*dth3*m3*sin(th2 + th3)^2*cos(th3)*sin(th1)^2)/5 + (Lc3*dth2^2*m3*cos(th2 + th3)*sin(th2 + th3)*cos(th1)^2*sin(th3))/5 + Lc3^2*dth1^2*m3*cos(th1)^2*cos(th2)*cos(th3)^2*sin(th2) + Lc3^2*dth1^2*m3*cos(th1)^2*cos(th2)^2*cos(th3)*sin(th3) + (Lc3*dth2^2*m3*cos(th2 + th3)*sin(th2 + th3)*sin(th1)^2*sin(th3))/5 + Lc3^2*dth1^2*m3*cos(th2)*cos(th3)^2*sin(th1)^2*sin(th2) - Lc3^2*dth1^2*m3*cos(th1)^2*cos(th2)*sin(th2)*sin(th3)^2 - Lc3^2*dth1^2*m3*cos(th1)^2*cos(th3)*sin(th2)^2*sin(th3) + Lc3^2*dth1^2*m3*cos(th2)^2*cos(th3)*sin(th1)^2*sin(th3) - Lc3^2*dth1^2*m3*cos(th2)*sin(th1)^2*sin(th2)*sin(th3)^2 - Lc3^2*dth1^2*m3*cos(th3)*sin(th1)^2*sin(th2)^2*sin(th3) - 2*Lc3^2*dth2*m3*cos(th2 + th3)*sin(th2 + th3)*cos(th1)^2*(dth2 + dth3) - 2*Lc3^2*dth3*m3*cos(th2 + th3)*sin(th2 + th3)*cos(th1)^2*(dth2 + dth3) - 2*Lc3^2*dth2*m3*cos(th2 + th3)*sin(th2 + th3)*sin(th1)^2*(dth2 + dth3) - 2*Lc3^2*dth3*m3*cos(th2 + th3)*sin(th2 + th3)*sin(th1)^2*(dth2 + dth3) + (Lc3*dth1^2*m3*cos(th1)^2*cos(th2)*sin(th2)*sin(th3))/5 + (Lc3*dth2*m3*cos(th2 + th3)^2*cos(th1)^2*cos(th3)*(dth2 + dth3))/5 + (Lc3*dth1^2*m3*cos(th2)*sin(th1)^2*sin(th2)*sin(th3))/5 + (Lc3*dth2*m3*cos(th2 + th3)^2*cos(th3)*sin(th1)^2*(dth2 + dth3))/5 - (Lc3*dth2*m3*sin(th2 + th3)^2*cos(th1)^2*cos(th3)*(dth2 + dth3))/5 - 2*Lc3^2*dth2*dth3*m3*cos(th2 + th3)*sin(th2 + th3)*cos(th1)^2 - (Lc3*dth2*m3*sin(th2 + th3)^2*cos(th3)*sin(th1)^2*(dth2 + dth3))/5 - 2*Lc3^2*dth2*dth3*m3*cos(th2 + th3)*sin(th2 + th3)*sin(th1)^2 + (Lc3*ddth2*m3*cos(th2 + th3)*sin(th2 + th3)*cos(th1)^2*cos(th3))/5 - (2*Lc3*dth2*m3*cos(th2 + th3)*sin(th2 + th3)*sin(th3)*(dth2 + dth3))/5 - (Lc3*dth2*dth3*m3*cos(th2 + th3)^2*cos(th1)^2*cos(th3))/5 + (2*Lc3*dth2*m3*cos(th2 + th3)*sin(th2 + th3)*cos(th1)^2*sin(th3)*(dth2 + dth3))/5 + (2*Lc3*dth2*m3*cos(th2 + th3)*sin(th2 + th3)*sin(th1)^2*sin(th3)*(dth2 + dth3))/5;
